simulink model "ee407_hw2_q3a"  (R2020a)
settings: Solver=FixedStepAuto  StartTime=0.0  StopTime=20  FixedStep=1e-5  RelTol=1e-3
undefined symbols (not defined in the file): n1, n2
settings Model: Creator=iky  LastModifiedBy=iky

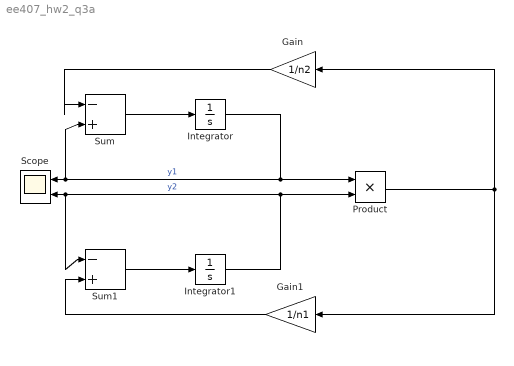
== system ee407_hw2_q3a ==
  Gain : Gain  Gain=1/n2
  Gain1 : Gain  Gain=1/n1
  Integrator : Integrator  InitialCondition=300
  Integrator1 : Integrator  InitialCondition=200
  Product : Product
  Scope : Scope  NumInputPorts=2
  Sum : Sum  Inputs=|-+
  Sum1 : Sum  Inputs=|-+
  wires:
  Integrator/1 -> Sum/2, Scope/1, Product/1  "y1"
  Sum/1 -> Integrator/1
  Product/1 -> Gain/1, Gain1/1
  Gain1/1 -> Sum1/2
  Gain/1 -> Sum/1
  Integrator1/1 -> Sum1/1, Scope/2, Product/2  "y2"
  Sum1/1 -> Integrator1/1
